simulink model "simple_EHGO_ASMC"  (R2023a)
settings: Solver=ode1  StartTime=0.0  StopTime=60  FixedStep=0.01  RelTol=1e-3
libraries: simulink x1, robotcorelib x1, dspsrcs4 x1
settings Model: Creator=Adan Daniel  LastModifiedBy=Adan Daniel
settings OptimizationCC: ReuseModelBlockBuffer=off

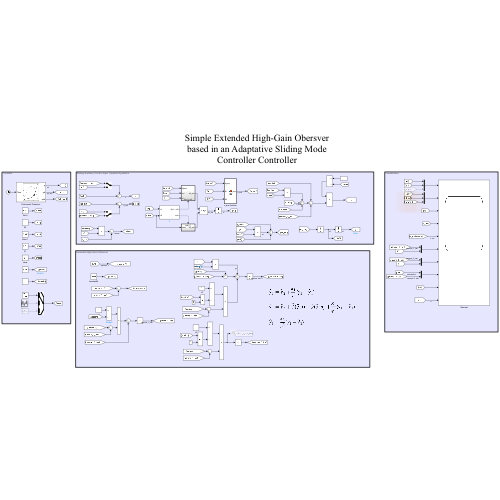
[thumbnail: Simulink's stored preview of the top-level diagram]
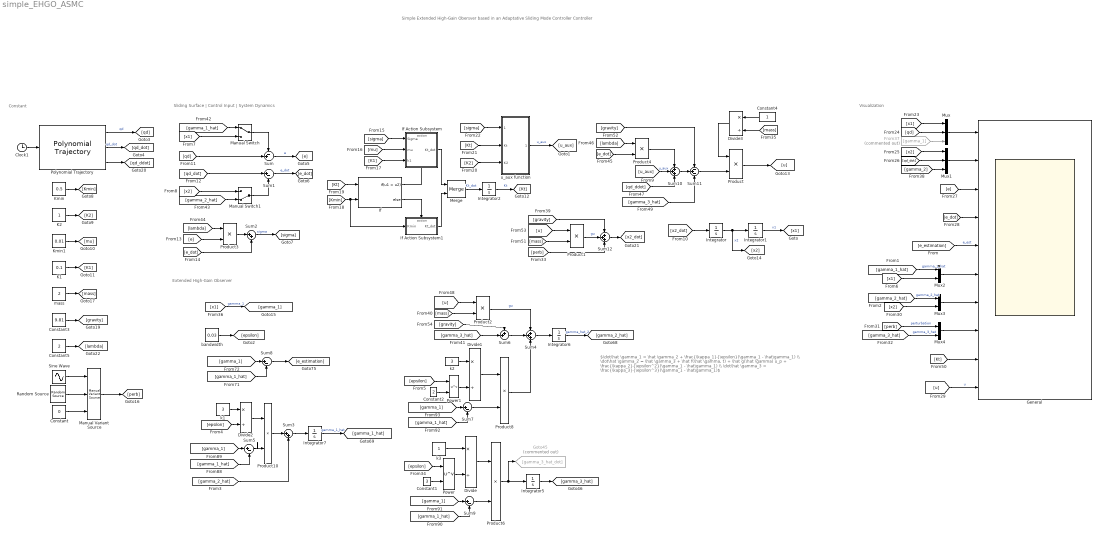
== system simple_EHGO_ASMC ==
  note: Extended High-Gain Observer
  note: Sliding Surface | Control Input | System Dynamics
  note: Constant
  note: Visualization
  note: Simple Extended High-Gain Obersver based in an Adaptative Sliding Mode Controller Controller
  note: $\dot\hat \gamma_1 = \hat \gamma_2 + \frac{\kappa_1}{\epsilon}(\gamma_1 - \hat\gamma_1) \\ \dot\hat \gamma_2 = \hat \gamma_3 + \hat f(\hat \gamma, t) + \hat g(\hat \gamma) u_p + \frac{\kappa_2}{\epsilon^2}(\gamma_1 - \hat\gamma_1) \\ \dot\hat \gamma_3 = \frac{\kappa_3}{\epsilon^3}(\gamma_1 - \hat\gamma_1)$
  Clock1 : Clock
  Constant : Constant  Value=0
  Constant1 : Constant  Value=3
  Constant2 : Constant  Value=2
  Constant3 : Constant  Value=9.81
  Constant4 : Constant
  Constant5 : Constant  Value=2
  Divide{,1..3} (4 alike) : Product  Inputs=*/
  From37 : From  Commented=on  GotoTag=gamma_1
  General : Scope  NumInputPorts=10
  Goto45 : Goto  Commented=on  GotoTag=gamma_3_hat_dot
  If : If  NumInputs=2  IfExpression=u1 > u2
  If Action Subsystem : Subsystem  TreatAsAtomicUnit=on
  If Action Subsystem1 : Subsystem  TreatAsAtomicUnit=on
  Integrator{,1..2,5..7} (6 alike) : Integrator
  K1 : Constant  Value=0.1
  K2 : Constant
  Kmin : Constant  Value=0.5
  Kmin1 : Constant  Value=0.01
  Manual Variant Source : simulink/Signal Routing/Manual Variant Source  NumChoices=3  LabelModeActiveChoice=V_1
  Manual Switch : ManualSwitch
  Manual Switch1 : ManualSwitch  CurrentSetting=0
  Merge : Merge
  Mux : Mux  Inputs=3
  Mux1 : Mux  Inputs=3
  Mux2 : Mux  Inputs=2
  Mux3 : Mux  Inputs=2
  Mux4 : Mux  Inputs=2
  Polynomial Trajectory : robotcorelib/Polynomial Trajectory  WaypointSource=Internal  Waypoints=[0, 2, 0, -2, 0, 1]  TimePoints=[0, 12, 24, 36, 48, 60]  TimeInterval=[ 1, 4 ]  Method=Cubic Polynomial  ParameterSource=Internal  VelocityBoundaryCondition=zeros( 1, 6 )  AccelerationBoundaryCondition=zeros( 2, 5 )  SimulateUsing=Interpreted execution
  Power : Math  Operator=pow
  Power1 : Math  Operator=pow
  Product{,1..4,6,8,10} (8 alike) : Product
  Random Source : dspsrcs4/Random Source  SrcType=Uniform  NormMethod=Ziggurat  CltLength=12  MinVal=-0.2  MaxVal=0.2  MeanVal=0  VarVal=1  RepMode=Not repeatable  rawSeed=1  IsInherit=off  SampMode=Discrete  SampTime=1  SampFrame=1  DataType=Double  OutComplex=Real  OutputFrames=off
  Sine Wave : Sin  Amplitude=0.2  Frequency=0.25  SampleTime=0
  Sum : Sum  Inputs=-+|
  Sum{1,5,7..9} (5 alike) : Sum  Inputs=|+-
  Sum10 : Sum  Inputs=+++
  Sum11 : Sum  Inputs=-+-
  Sum12 : Sum  Inputs=+++
  Sum2 : Sum  Inputs=|++
  Sum3 : Sum  Inputs=|++
  Sum4 : Sum  Inputs=+++
  Sum6 : Sum  Inputs=++|
  bandwidth : Constant  Value=0.03
  k1 : Constant  Value=3
  k2 : Constant  Value=3
  k3 : Constant
  mass : Constant  Value=2
  u_aux function : MATLAB Function  TreatAsAtomicUnit=on
  wires:
  Integrator1/1 -> [x1]  "x1"
  Integrator/1 -> [x2], Integrator1/1  "x2"
  Sum1/1 -> [e_dot]  "e_dot"
  Mux/1 -> General/1
  Product3/1 -> Sum2/1
  u_aux function/1(u_aux) -> [u_aux]  "u_aux"
  Merge/1 -> Integrator2/1  "Kt_dot"
  If/1 -> If Action Subsystem/Action
  If/2 -> If Action Subsystem1/Action
  If Action Subsystem/1(Kt_dot) -> Merge/1
  If Action Subsystem1/1(Kt_dot) -> Merge/2
  [x2_dot] -> Integrator/1
  Clock1/1 -> Polynomial Trajectory/1
  Polynomial Trajectory/3 -> [qd_ddot]
  Sum5/1 -> Product10/2
  Sum3/1 -> Integrator7/1
  [gamma_1_hat] -> Sum5/2
  k1/1 -> Divide2/1
  Product10/1 -> Sum3/1
  Integrator7/1 -> [gamma_1_hat]  "gamma_1_hat"
  [epsilon] -> Divide2/2
  [gamma_1] -> Sum5/1
  Divide2/1 -> Product10/1
  [gamma_2_hat] -> Sum3/2
  [gamma_1_hat] -> Sum7/2
  [gamma_1] -> Sum7/1
  Constant2/1 -> Power1/2
  [epsilon] -> Power1/1
  [gamma_1] -> Sum8/1
  Sum7/1 -> Product8/2
  Power1/1 -> Divide1/2
  [gamma_1_hat] -> Sum8/2
  Sum8/1 -> [e_estimation]
  k2/1 -> Divide1/1
  Integrator6/1 -> [gamma_2_hat]  "gamma_hat_2"
  Divide1/1 -> Product8/1
  Sum4/1 -> Integrator6/1
  Product8/1 -> Sum4/3
  [e_estimation] -> General/5  "e_est"
  [gamma_1_hat] -> Mux2/1  "gamma_1_hat"
  [gamma_2_hat] -> Mux3/1  "gamma_2_hat"
  bandwidth/1 -> [epsilon]
  Mux2/1 -> General/6
  [x1] -> Mux2/2
  Mux3/1 -> General/7
  [x1] -> Manual Switch/2
  [x2] -> Manual Switch1/1
  [qd] -> Mux/2
  Polynomial Trajectory/1 -> [qd]  "qd"
  Polynomial Trajectory/2 -> [qd_dot]  "qd_dot"
  [qd] -> Sum/2
  [qd_dot] -> Sum1/1
  Sum/1 -> [e]  "e"
  [e] -> Product3/2
  [e_dot] -> Sum2/2
  Sum2/1 -> [sigma]  "sigma"
  Kmin/1 -> [Kmin]
  K2/1 -> [K2]
  [sigma] -> If Action Subsystem/1(Sigma)
  Kmin1/1 -> [mu]
  K1/1 -> [K1]
  [mu] -> If Action Subsystem/2(mu)
  [K1] -> If Action Subsystem/3(k1)
  [Kmin] -> If/2, If Action Subsystem1/1(Kmin)
  Integrator2/1 -> [Kt]  "Kt"
  [Kt] -> If/1
  [sigma] -> u_aux function/1(sigma)
  [Kt] -> u_aux function/2(Kt)
  [K2] -> u_aux function/3(K2)
  [x1] -> Mux/1
  [qd_dot] -> Mux1/2
  [x2] -> Mux1/1
  Mux1/1 -> General/2
  [e] -> General/3
  [e_dot] -> General/4
  [x1] -> [gamma_1]  "gamma_1"
  [x2] -> Mux3/2
  [perb] -> Mux4/1  "perturbation"
  Manual Variant Source/1 -> [perb]
  Sine Wave/1 -> Manual Variant Source/1
  Random Source/1 -> Manual Variant Source/2
  [gamma_1_hat] -> Sum9/2
  [gamma_1] -> Sum9/1
  Sum9/1 -> Product6/2
  Power/1 -> Divide/2
  Product6/1 -> Integrator5/1, Goto45/1
  Integrator5/1 -> [gamma_3_hat]
  Divide/1 -> Product6/1
  Constant1/1 -> Power/2
  k3/1 -> Divide/1
  [epsilon] -> Power/1
  Mux4/1 -> General/8
  [gamma_3_hat] -> Mux4/2  "gamma_3_hat"
  mass/1 -> [mass]
  [u_aux] -> Sum10/2  "u_aux"
  [mass] -> Divide3/2
  Product2/1 -> Sum4/1  "gu"
  [u] -> Product2/1
  [mass] -> Product2/2
  From37/1 -> Mux/3
  [gamma_2] -> Mux1/3
  Constant/1 -> Manual Variant Source/3
  Manual Switch/1 -> Sum/1
  Manual Switch1/1 -> Sum1/2
  [gamma_2_hat] -> Manual Switch1/2
  [gamma_1_hat] -> Manual Switch/1
  Constant3/1 -> [gravity]
  [lambda] -> Product3/1
  [e_dot] -> Product4/2
  [lambda] -> Product4/1
  Product4/1 -> Sum10/1
  [qd_ddot] -> Sum10/3
  Constant4/1 -> Divide3/1
  Divide3/1 -> Product/1
  Sum10/1 -> Sum11/2
  Sum11/1 -> Product/2
  Product/1 -> [u]
  [gamma_3_hat] -> Sum11/3
  [Kt] -> General/9
  Constant5/1 -> [lambda]
  [u] -> General/10  "u"
  [u] -> Product1/1
  [mass] -> Product1/2
  Sum12/1 -> [x2_dot]
  Product1/1 -> Sum12/2  "gu"
  [gravity] -> Sum12/1
  [perb] -> Sum12/3
  [gravity] -> Sum11/1
  [gamma_3_hat] -> Sum6/2
  Sum6/1 -> Sum4/2
  [gravity] -> Sum6/1

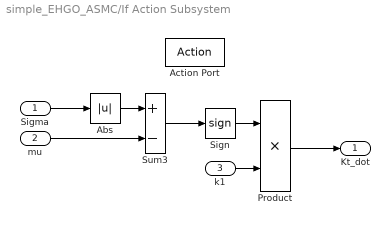
== system simple_EHGO_ASMC/If Action Subsystem ==
  Sigma : Inport
  mu : Inport  Port=2
  k1 : Inport  Port=3
  Action Port : ActionPort  ActionPortLabel=if(u1 > u2)
  Abs : Abs  SaturateOnIntegerOverflow=off
  Product : Product
  Sign : Signum
  Sum3 : Sum  Inputs=+-
  Kt_dot : Outport
  wires:
  Sign/1 -> Product/1
  mu/1 -> Sum3/2
  Sum3/1 -> Sign/1
  Abs/1 -> Sum3/1
  Product/1 -> Kt_dot/1
  Sigma/1 -> Abs/1
  k1/1 -> Product/2

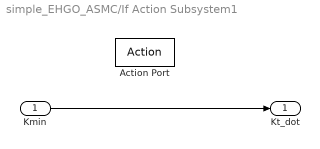
== system simple_EHGO_ASMC/If Action Subsystem1 ==
  Kmin : Inport
  Action Port : ActionPort  ActionPortLabel=else
  Kt_dot : Outport
  wires:
  Kmin/1 -> Kt_dot/1

== matlab function simple_EHGO_ASMC/u_aux function ==
  data: sigma input; u_aux output; Kt input; K2 input
function u_aux = fcn(sigma, Kt, K2)

u_aux = - Kt * (abs(sigma) ^ (0.5)) * sign(sigma) - K2 * sigma;
u_aux = -u_aux;
